simulink model "Ex1_inertia_2020a"  (R2024a)
settings: Solver=VariableStepAuto  StartTime=0.0  StopTime=50  MaxStep=1e-4  RelTol=1e-3
values from neighbouring files (symbols this model uses):
  fixed_kdroop = 0.05    [Ex1_parameters.m]
  fixed_tau_gen = 5    [Ex1_parameters.m]
  H = Ho*0.5    (= 2.5)    [Ex1_parameters.m]
  kdroop = 0.05    [Ex1_parameters.m]
  M = J*w    (= 7957747.15459)    [Ex1_parameters.m]
  Sb = 500e6    (= 500000000)    [Ex1_parameters.m]
  sp = 1/kdroop*Sb/w    (= 31830988.6184)    [Ex1_parameters.m]
  tau_gen = 5    [Ex1_parameters.m]
  w = 2*pi*50    (= 314.159265359)    [Ex1_parameters.m]
settings Model: Creator=eprieto  LastModifiedBy=citcea
settings SolverCC: AlgebraicLoopSolver=TrustRegion
settings DebuggingCC: UnconnectedInputMsg=warning  UnconnectedOutputMsg=warning  UnconnectedLineMsg=warning
settings ModelReferenceCC: EnableRefExpFcnMdlSchedulingChecks=on
settings RTWCC: GPUComputeCapability=3.5

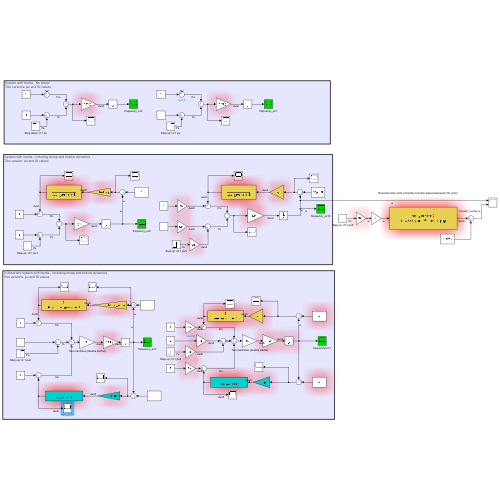
[thumbnail: Simulink's stored preview of the top-level diagram]
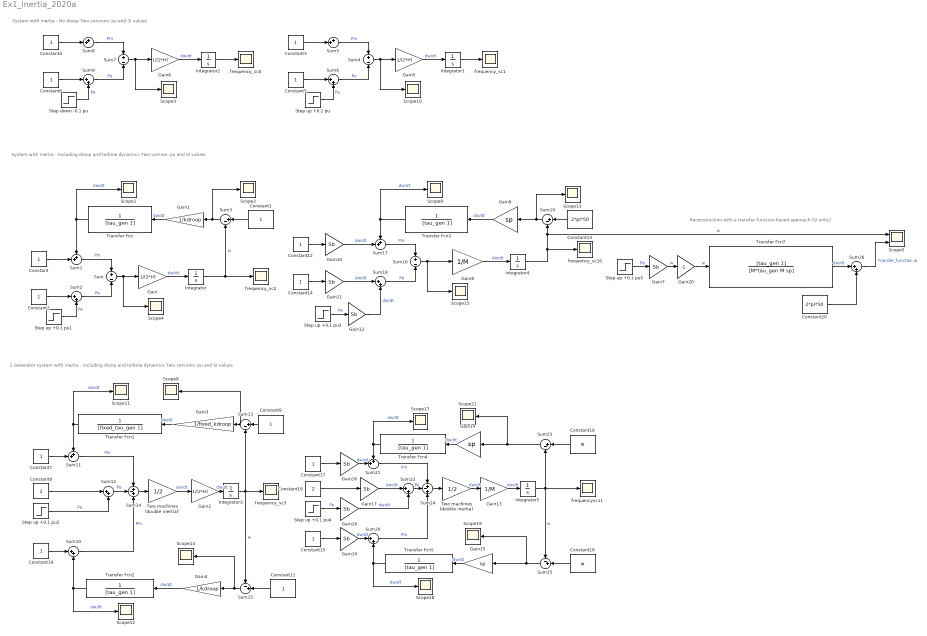
== system Ex1_inertia_2020a ==
  note: Reconstruction with a transfer-function-based approach (SI units)
  note: 2 Generator system with inertia - Including droop and turbine dynamics
      | Two versions: pu and SI values
  note: System with inertia - Including droop and turbine dynamics
      | Two version: pu and SI values
  note: System with inertia - No droop
      | Two versions: pu and SI values
  Constant{,1..8,10..12,14..15,17} (15 alike) : Constant
  Constant13 : Constant  Value=2*pi*50
  Constant16 : Constant  Value=w
  Constant18 : Constant  Value=w
  Constant19 : Constant  Value=2
  Constant20 : Constant  Value=2*pi*50
  Constant9 : Constant  Value=2
  Gain{,2,5..6} (4 alike) : Gain  Gain=1/(2*H)
  Gain1 : Gain  Gain=1/kdroop
  Gain{7,10..12,16..19} (8 alike) : Gain  Gain=Sb
  Gain13 : Gain  Gain=1/M
  Gain14 : Gain  Gain=sp
  Gain15 : Gain  Gain=sp
  Gain20 : Gain  Gain=-1
  Gain3 : Gain  Gain=1/fixed_kdroop
  Gain4 : Gain  Gain=1/kdroop
  Gain8 : Gain  Gain=1/M
  Gain9 : Gain  Gain=sp
  Integrator{,1..3} (4 alike) : Integrator  InitialCondition=1
  Integrator4 : Integrator  InitialCondition=2*pi*50
  Integrator5 : Integrator  InitialCondition=w
  Scope{1..4,8..15,17..19,21} (16 alike) : Scope
  Scope5 : Scope  NumInputPorts=2
  Step down -0.1 pu : Step  After=-0.1  SampleTime=0
  Step up +0.1 pu{,1,3,5} (4 alike) : Step  After=0.1  SampleTime=0
  Step up +0.1 pu2 : Step  After=0.2  SampleTime=0
  Step up +0.1 pu4 : Step  After=0.2  SampleTime=0
  Sum{,4,7,16} (4 alike) : Sum  Inputs=+-
  Sum{1,5,8,11,17,21} (6 alike) : Sum  Inputs=++|
  Sum{2,6,9..10,12,18,20,22,26} (9 alike) : Sum  Inputs=|++
  Sum{3,13,19,23} (4 alike) : Sum  Inputs=|+-
  Sum14 : Sum  Inputs=+-+
  Sum15 : Sum  Inputs=-+|
  Sum24 : Sum  Inputs=+-+
  Sum25 : Sum  Inputs=-+|
  Transfer Fcn{,2..5} (5 alike) : TransferFcn  Denominator=[tau_gen 1]
  Transfer Fcn1 : TransferFcn  Denominator=[fixed_tau_gen 1]
  Transfer Fcn7 : TransferFcn  Numerator=[tau_gen 1]  Denominator=[M*tau_gen M sp]
  Two machines (double inertia) : Gain  Gain=1/2
  Two machines (double inertia)' : Gain  Gain=1/2
  frequency_sc{0..3,10} (5 alike) : Scope
  frequencysc11 : Scope
  wires:
  Sum1/1 -> Sum/1  "Pm"
  Sum2/1 -> Sum/2  "Pe"
  Sum/1 -> Scope4/1, Gain/1
  Gain/1 -> Integrator/1  "dw/dt"
  Step up +0.1 pu1/1 -> Sum2/2  "Pe"
  Constant/1 -> Sum1/2
  Constant2/1 -> Sum2/1
  Constant1/1 -> Sum3/1
  Sum3/1 -> Gain1/1, Scope2/1
  Gain1/1 -> Transfer Fcn/1  "dw/dt"
  Transfer Fcn/1 -> Sum1/1, Scope1/1  "dw/dt"
  Integrator/1 -> Sum3/2, frequency_sc2/1  "w"
  Step up +0.1 pu/1 -> Sum6/2  "Pe"
  Constant3/1 -> Sum5/2
  Sum6/1 -> Sum4/2  "Pe"
  Gain5/1 -> Integrator1/1  "dw/dt"
  Sum5/1 -> Sum4/1  "Pm"
  Sum4/1 -> Scope10/1, Gain5/1
  Constant5/1 -> Sum6/1
  Integrator1/1 -> frequency_sc1/1
  Integrator2/1 -> frequency_sc0/1
  Constant6/1 -> Sum9/1
  Sum7/1 -> Gain6/1, Scope3/1
  Sum8/1 -> Sum7/1  "Pm"
  Gain6/1 -> Integrator2/1  "dw/dt"
  Sum9/1 -> Sum7/2  "Pe"
  Constant4/1 -> Sum8/2
  Step down -0.1 pu/1 -> Sum9/2  "Pe"
  Integrator3/1 -> Sum13/2, Sum15/1, frequency_sc3/1  "w"
  Transfer Fcn1/1 -> Scope11/1, Sum11/1  "dw/dt"
  Gain3/1 -> Transfer Fcn1/1  "dw/dt"
  Sum13/1 -> Gain3/1, Scope8/1
  Constant8/1 -> Sum13/1
  Constant9/1 -> Sum12/1
  Constant7/1 -> Sum11/2
  Gain2/1 -> Integrator3/1  "dw/dt"
  Sum12/1 -> Sum14/2  "Pe"
  Sum11/1 -> Sum14/1  "Pm"
  Step up +0.1 pu2/1 -> Sum12/2  "Pe"
  Sum14/1 -> Two machines (double inertia)'/1
  Sum10/1 -> Sum14/3  "Pm"
  Constant10/1 -> Sum10/1
  Constant11/1 -> Sum15/2
  Sum15/1 -> Gain4/1, Scope14/1
  Gain4/1 -> Transfer Fcn2/1  "dw/dt"
  Transfer Fcn2/1 -> Scope12/1, Sum10/2  "dw/dt"
  Two machines (double inertia)'/1 -> Gain2/1  "dw/dt"
  Sum18/1 -> Sum16/2  "Pe"
  Transfer Fcn3/1 -> Sum17/1, Scope9/1  "dw/dt"
  Gain9/1 -> Transfer Fcn3/1  "dw/dt"
  Constant14/1 -> Gain11/1
  Constant13/1 -> Sum19/1
  Gain8/1 -> Integrator4/1  "dw/dt"
  Constant12/1 -> Gain10/1
  Step up +0.1 pu3/1 -> Gain12/1  "Pe"
  Sum16/1 -> Scope15/1, Gain8/1
  Sum17/1 -> Sum16/1  "Pm"
  Sum19/1 -> Scope13/1, Gain9/1
  Integrator4/1 -> frequency_sc10/1, Scope5/1, Sum19/2  "w"
  Gain10/1 -> Sum17/2  "dw/dt"
  Gain11/1 -> Sum18/1  "dw/dt"
  Gain12/1 -> Sum18/2  "dw/dt"
  Constant16/1 -> Sum25/2
  Integrator5/1 -> Sum23/2, Sum25/1, frequencysc11/1  "w"
  Sum21/1 -> Sum24/1  "Pm"
  Constant15/1 -> Gain19/1
  Constant18/1 -> Sum23/1
  Transfer Fcn4/1 -> Scope17/1, Sum21/1  "dw/dt"
  Gain14/1 -> Transfer Fcn4/1  "dw/dt"
  Constant17/1 -> Gain16/1
  Step up +0.1 pu4/1 -> Gain18/1  "Pe"
  Gain13/1 -> Integrator5/1  "dw/dt"
  Sum23/1 -> Scope21/1, Gain14/1
  Sum20/1 -> Sum24/3  "Pm"
  Sum22/1 -> Sum24/2  "Pe"
  Transfer Fcn5/1 -> Scope18/1, Sum20/2  "dw/dt"
  Two machines (double inertia)/1 -> Gain13/1  "dw/dt"
  Sum25/1 -> Scope19/1, Gain15/1
  Constant19/1 -> Gain17/1
  Sum24/1 -> Two machines (double inertia)/1
  Gain15/1 -> Transfer Fcn5/1  "dw/dt"
  Gain16/1 -> Sum21/2  "dw/dt"
  Gain17/1 -> Sum22/1  "dw/dt"
  Gain18/1 -> Sum22/2  "dw/dt"
  Gain19/1 -> Sum20/1  "dw/dt"
  Step up +0.1 pu5/1 -> Gain7/1  "Pe"
  Gain7/1 -> Gain20/1  "w"
  Sum26/1 -> Scope5/2  "Transfer_function w"
  Constant20/1 -> Sum26/2
  Transfer Fcn7/1 -> Sum26/1  "dw/dt"
  Gain20/1 -> Transfer Fcn7/1  "w"
